simulink model "planmodel2023"  (R2023b)
settings: Solver=ode4  StartTime=0.0  StopTime=200  FixedStep=0.001  RelTol=1e-3
values from neighbouring files (symbols this model uses):
  a0 = 340.294    [plan.m]    (also in plan.mat)
  b_ref = 2.0    (= 2)    [plan.m]    (also in plan.mat)
  c_gear = [0.8e4, 1.4e4, 1.4e4]    [plan.m]    (also in plan.mat = [8000 14000 14000])
  c_lat = [1.4e4, 2.2e4, 2.2e4]    [plan.m]    (also in plan.mat = [14000 22000 22000])
  c_ref = 0.9    [plan.m]    (also in plan.mat)
  c_roll = [0.020, 0.018, 0.018]    [plan.m]    (also in plan.mat = [0.02 0.018 0.018])
  CD0 = 0.045    [plan.m]    (also in plan.mat)
  CL0 = 0.083    [plan.m]    (also in plan.mat)
  CLa = 2.50    (= 2.5)    [plan.m]    (also in plan.mat = 3.8)
  Clb = -0.08    [plan.m]    (also in plan.mat)
  Clda = 0.20    (= 0.2)    [plan.m]    (also in plan.mat = -0.2)
  CLde = 0.25    [plan.m]    (also in plan.mat = 0.28)
  Clp = -0.70    (= -0.7)    [plan.m]    (also in plan.mat)
  CLq = 3.00    (= 3)    [plan.m]    (also in plan.mat = 4.5)
  Clr = 0    [plan.m]    (also in plan.mat = 0.08)
  Cm0 = 0.112    [plan.m]    (also in plan.mat = 0.06)
  Cma = -0.8    [plan.m]    (also in plan.mat)
  Cmde = 0.90    (= 0.9)    [plan.m]    (also in plan.mat = -0.9)
  Cmq = -18.0    (= -18)    [plan.m]    (also in plan.mat)
  Cnb = -0.25    [plan.m]    (also in plan.mat = 0.25)
  Cndr = 0.15    [plan.m]    (also in plan.mat = -0.15)
  Cnp = 0    [plan.m]    (also in plan.mat = -0.04)
  Cnr = -0.45    [plan.m]    (also in plan.mat)
  CSb = -0.8    [plan.m]    (also in plan.mat = -0.7)
  CSdr = 0.18    [plan.m]    (also in plan.mat)
  CSr = 0.15    [plan.m]    (also in plan.mat = 0.12)
  D0 = 800    [plan.m]    (also in plan.mat)
  da_max = 25    [plan.m]    (also in plan.mat)
  da_min = -da_max    (= -25)    [plan.m]    (also in plan.mat)
  de_max = 25    [plan.m]    (also in plan.mat)
  de_min = -de_max    (= -25)    [plan.m]    (also in plan.mat)
  DH = pi / 180    (= 0.0174532925199)    [plan.m]    (also in plan.mat)
  dr_max = 25    [plan.m]    (also in plan.mat)
  dr_min = -dr_max    (= -25)    [plan.m]    (also in plan.mat)
  g = 9.80665    [plan.m]    (also in plan.mat)
  gamma0 = 0.0    (= 0)    [plan.m]
  ground_y = 0.0    (= 0)    [plan.m]
  HD = 180 / pi    (= 57.2957795131)    [plan.m]    (also in plan.mat)
  Ixx = 120.0    (= 120)    [plan.m]    (also in plan.mat)
  Iyy = 480.0    (= 480)    [plan.m]    (also in plan.mat)
  Izz = 520.0    (= 520)    [plan.m]    (also in plan.mat)
  K = 0.080    (= 0.08)    [plan.m]    (also in plan.mat = 0.12)
  K_alpha = 7.67884615385    [plan.mat]
  k_gear = [1.0e5, 3.0e5, 3.0e5]    [plan.m]    (also in plan.mat = [100000 300000 300000])
  k_theta0 = 0.0    (= 0)    [plan.m]
  Kb_to_wy = 10.6510416667    [plan.mat]
  Kn_pitch = 0.117046638908    [plan.mat]
  Kn_to_beta = 0.461367696223    [plan.mat]
  Kw_pitch = -0.524061476442    [plan.mat]
  Kw_to_dr = -1.30612244898    [plan.mat]
  m = 600.0    (= 600)    [plan.m]    (also in plan.mat)
  mu_brake = [0.0, 0.55, 0.55]    [plan.m]    (also in plan.mat = [0 0.55 0.55])
  omigax0 = 0    [plan.m]
  omigay0 = 0    [plan.m]
  omigaz0 = 0    [plan.m]
  psi0 = 0.3/57.3    (= 0.00523560209424)    [plan.m]    (also in plan.mat = 0)
  r_left_b = r_gear_b(:,2)    [plan.m]    (also in plan.mat = [-0.333333333333 -0.8 0.65])
  r_nose_b = r_gear_b(:,1)    [plan.m]    (also in plan.mat = [2 0 0.65])
  r_right_b = r_gear_b(:,3)    [plan.m]    (also in plan.mat = [-0.333333333333 0.8 0.65])
  rho0 = 1.225    [plan.m]    (also in plan.mat)
  S_ref = 1.2    [plan.m]    (also in plan.mat)
  v_eps = 0.20    (= 0.2)    [plan.m]    (also in plan.mat)
  V_min = 1    [plan.m]    (also in plan.mat = 3)
  V_test = 200    [plan.mat]
  Vx0_b = 0.0    (= 0)    [plan.m]
  Vy0_b = 0.0    (= 0)    [plan.m]
  Vz0_b = 0.0    (= 0)    [plan.m]
  wheel_radius = 0.18    [plan.m]    (also in plan.mat)
  WOW_on = 0.000    (= 0)    [plan.m]    (also in plan.mat)
  Xg0 = 0.0    (= 0)    [plan.m]    (also in plan.mat)
  Yg0 = ground_y + wheel_radius - r_gear_b(2,1) - static_deflection    [plan.m]    (also in plan.mat = 0)
  Zg0 = 1.0    (= 1)    [plan.m]    (also in plan.mat = -0.8215943)
libraries: matrix_library x18, slpidlib x1
(part 3 of 3)

== matlab function planmodel2023/6DOF-MODEL/动力学/v在体系下的分量/MATLAB Function ==
  data: alpha input; R_wind_b output; beta input
 function R_wind_b = wind2body(alpha, beta)
T1 = [cos(beta), 0, -sin(beta);
       0, 1, 0;
       sin(beta), 0, cos(beta)];
T2 = [cos(alpha), sin(alpha), 0;
       -sin(alpha), cos(alpha), 0;
       0, 0, 1];
R_wind_b = T2*T1;

== matlab function planmodel2023/6DOF-MODEL/动力学/v在体系下的分量/MATLAB Function1 ==
  data: gamma input; R_gb output; theta input; psi input
function R_gb = ground2body(gamma, theta, psi)
    T1=[cos(psi), 0 ,-sin(psi);...
          0     , 1 ,    0   ;...
        sin(psi), 0 ,cos(psi);];%绕y偏航
    T2=[cos(theta),sin(theta),0;...
        -sin(theta),cos(theta),0;...
          0        , 0 ,       1;];%绕z俯仰角
    T3=[1,0,0;...
        0,cos(gamma),sin(gamma);...
        0,-sin(gamma),cos(gamma);];%绕x滚转角

   R_gb=T3*T2*T1;

== matlab function planmodel2023/6DOF-MODEL/动力学/起落架模型/法向支反力/MATLAB Function1 ==
  data: gamma input; R_gb output; theta input; psi input
function R_gb = ground2body(gamma, theta, psi)
    T1=[cos(psi), 0 ,-sin(psi);...
          0     , 1 ,    0   ;...
        sin(psi), 0 ,cos(psi);];%绕y偏航
    T2=[cos(theta),sin(theta),0;...
        -sin(theta),cos(theta),0;...
          0        , 0 ,       1;];%绕z俯仰角
    T3=[1,0,0;...
        0,cos(gamma),sin(gamma);...
        0,-sin(gamma),cos(gamma);];%绕x滚转角

   R_gb=T3*T2*T1;

== matlab function planmodel2023/6DOF-MODEL/动力学/起落架模型/纵向力/Subsystem/MATLAB Function1 ==
  data: gamma input; R_gb output; theta input; psi input
function R_gb = ground2body(gamma, theta, psi)
    T1=[cos(psi), 0 ,-sin(psi);...
          0     , 1 ,    0   ;...
        sin(psi), 0 ,cos(psi);];%绕y偏航
    T2=[cos(theta),sin(theta),0;...
        -sin(theta),cos(theta),0;...
          0        , 0 ,       1;];%绕z俯仰角
    T3=[1,0,0;...
        0,cos(gamma),sin(gamma);...
        0,-sin(gamma),cos(gamma);];%绕x滚转角

   R_gb=T3*T2*T1;

== matlab function planmodel2023/6DOF-MODEL/动力学/起落架模型/纵向力/Subsystem/前轮滚动方向向量 ==
  data: Cbg input; eg_long output; eb_long input
function eg_long= project_long(Cbg,eb_long)

e_y=[0;1;0];
P_g=eye(3)-e_y*e_y';
eg_long=P_g*Cbg*eb_long;
eg_long=eg_long/norm(eg_long);

== matlab function planmodel2023/6DOF-MODEL/动力学/起落架模型/纵向力/Subsystem/主轮滚动方向向量 ==
  data: Cbg input; eg_long output; eb_long input
function eg_long= project_long(Cbg,eb_long)


e_y=[0;1;0];
P_g=eye(3)-e_y*e_y';

eg_long=P_g*Cbg*eb_long;
eg_long=eg_long/norm(eg_long);
